simulink model "SguanFOC"  (R2025a)
settings: Solver=FixedStepAuto  StartTime=0.0  StopTime=5  FixedStep=0.00001  RelTol=1e-3
InitFcn:
  | T = 0.0001;
  | VBUS = 12;
  | 
  | Wc = 10;
  | Ws = 50;
undefined symbols (not defined in the file): Down, Up
libraries: eePwmGenerator x3, spsDCVoltageSourceLib x1, spsPermanentMagnetSynchronousMachineLib x1, spsSawtoothGeneratorLib x1, spsUniversalBridgeLib x1, spspowerguiLib x1
settings Model: Creator=星必尘Sguan  LastModifiedBy=星必尘Sguan
settings SFSimCC: SimCustomHeaderCode="#include \"SVPWM.h\""  SimUserSources=SVPWM.c

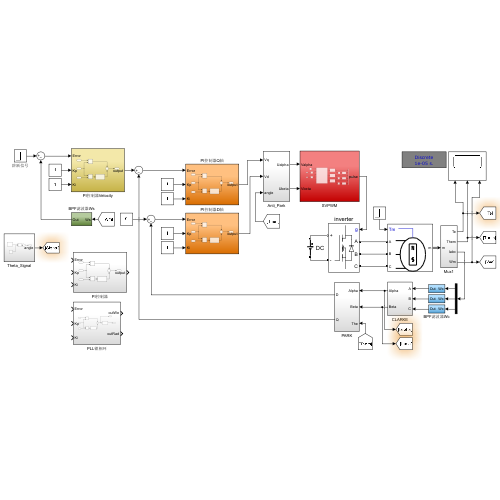
[thumbnail: Simulink's stored preview of the top-level diagram]
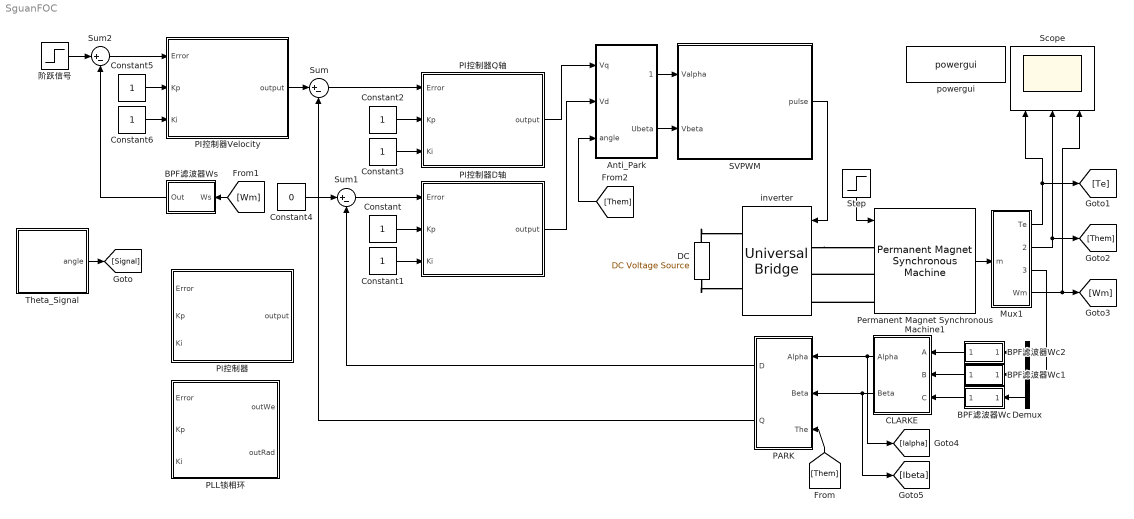
== system SguanFOC ==
  Anti_Park : Subsystem
  BPF滤波器Wc : Subsystem
  BPF滤波器Wc1 : Subsystem
  BPF滤波器Wc2 : Subsystem
  BPF滤波器Ws : Subsystem
  CLARKE : Subsystem
  Constant{,1..3,5..6} (6 alike) : Constant
  Constant4 : Constant  Value=0
  DC : spsDCVoltageSourceLib/DC Voltage Source  Amplitude=VBUS  Measurements=Voltage
  Demux : Demux  Outputs=3
  Mux1 : Subsystem
  PARK : Subsystem
  PI控制器 : Subsystem
  PI控制器D轴 : Subsystem
  PI控制器Q轴 : Subsystem
  PI控制器Velocity : Subsystem
  PLL锁相环 : Subsystem
  Permanent Magnet Synchronous Machine1 : spsPermanentMagnetSynchronousMachineLib/Permanent Magnet Synchronous Machine  NbPhases=3  FluxDistribution=Sinusoidal  RotorType=Salient-pole  MechanicalLoad=Torque Tm  PresetModel=No  ShowDetailedParameters=on  MeasurementBus=off  Resistance=0.958  Inductance=8.5e-3  dqInductances=[5.25e-3,12e-3]  La=0.000835  MachineConstant=Flux linkage established by magnets (V.s)  Flux=0.0234  VoltageCst=16.9772  TorqueCst=0.1404  Flat=120  Mechanical=[0.00025 0 4]  PolePairs=3  InitialConditions=[0,0, 0,0]  InitialConditions5ph=[0 0 0 0 0 0]  RefAngle=Aligned with phase A axis (original Park)  IterativeDiscreteModel=Trapezoidal non iterative  TsBlock=-1  TsPowergui=0
  SVPWM : Subsystem
  Scope : Scope  NumInputPorts=3
      settings: ActiveDisplayYMinimum=-17.449565790069414  ActiveDisplayYMaximum=24.577855803107717
  Step : Step  Time=0  After=0  SampleTime=0
  Sum : Sum  Inputs=|+-
  Sum1 : Sum  Inputs=|+-
  Sum2 : Sum  Inputs=|+-
  Theta_Signal : Subsystem
  inverter : spsUniversalBridgeLib/Universal Bridge  Arms=3  SnubberResistance=100  SnubberCapacitance=1e-5  Device=MOSFET / Diodes  Ron=1e-3  Lon=0  ForwardVoltages="[  0  0  ]"  ForwardVoltage=0  GTOparameters=[ 10e-6 , 20e-6 ]  IGBTparameters=[ 1e-6 , 2e-6 ]  Measurements=None  Measurements_2=None  converterType=Rectifier
  powergui : spspowerguiLib/powergui  SimulationMode=Discrete  SampleTime=1e-5  frequency=60  Iterations=50  frequencyindice=0  Pbase=100e6  ErrMax=1e-4  UnitsV=kV  UnitsW=MW  buscounter=0  FunctionMessages=off  echomessages=off  EnableUseOfTLC=off  CurrentSourceSwitches=off  DisableSnubberDevices=off  DisableRonSwitches=off  DisableVfSwitches=off  DisplayEquations=off  AutomaticDiscreteSolvers=off  SolverType=Tustin/Backward Euler (TBE)  Interpol=off  ExternalGateDelay=off  methode=off  Ts=0  x0status=blocks  SPID=off  SwTol=0  HookPort=off  NonlinearTolerance=1e-4  nMaxIteration=100  ContinueOnMaxIteration=off  RestoreLinks=warning  ResistiveCurrentMeasurement=off  Frange=[0:2:500]  Ylog=off  Xlog=on  ShowGrid=off  save=off  variable=ZData  structure=0  ZoomFFT=on  StartTime=0.0  cycles=1  DisplayStyle=1  fundamental=60  FreqAxis=off  MaxFrequency=1000  frequencyindicesteady=1  RmsSteady=1  display=off
  阶跃信号 : Step  Time=3  After=72  SampleTime=1e-5
  wires:
  Step/1 -> Permanent Magnet Synchronous Machine1/1
  Permanent Magnet Synchronous Machine1/1 -> Mux1/1(m)
  Anti_Park/1(Ualpha) -> SVPWM/1(Valpha)
  Anti_Park/2(Ubeta) -> SVPWM/2(Vbeta)
  SVPWM/1(pulse) -> inverter/1
  Mux1/3(Iabc) -> Demux/1
  Theta_Signal/1(angle) -> [Signal]
  PI控制器Q轴/1(output) -> Anti_Park/1(Vq)
  PI控制器D轴/1(output) -> Anti_Park/2(Vd)
  Constant/1 -> PI控制器D轴/2(Kp)
  Constant1/1 -> PI控制器D轴/3(Ki)
  Constant2/1 -> PI控制器Q轴/2(Kp)
  Constant3/1 -> PI控制器Q轴/3(Ki)
  Sum/1 -> PI控制器Q轴/1(Error)
  PI控制器Velocity/1(output) -> Sum/1
  Sum1/1 -> PI控制器D轴/1(Error)
  Demux/1 -> BPF滤波器Wc2/1(Wc)
  Demux/2 -> BPF滤波器Wc1/1(Wc)
  Demux/3 -> BPF滤波器Wc/1(Wc)
  CLARKE/1(Alpha) -> PARK/1(Alpha), [Ialpha]
  CLARKE/2(Beta) -> PARK/2(Beta), [Ibeta]
  Mux1/1(Te) -> [Te], Scope/1
  Mux1/2(Them) -> [Them], Scope/2
  Mux1/4(Wm) -> [Wm], Scope/3
  [Them] -> PARK/3(The)
  PARK/1(D) -> Sum1/2
  PARK/2(Q) -> Sum/2
  Constant4/1 -> Sum1/1
  阶跃信号/1 -> Sum2/1
  Sum2/1 -> PI控制器Velocity/1(Error)
  [Wm] -> BPF滤波器Ws/1(Ws)
  Constant5/1 -> PI控制器Velocity/2(Kp)
  Constant6/1 -> PI控制器Velocity/3(Ki)
  [Them] -> Anti_Park/3(angle)
  BPF滤波器Ws/1(Out) -> Sum2/2
  BPF滤波器Wc2/1(Out) -> CLARKE/1(A)
  BPF滤波器Wc1/1(Out) -> CLARKE/2(B)
  BPF滤波器Wc/1(Out) -> CLARKE/3(C)
  connections:
  DC/RConn1 -- inverter/RConn1
  DC/LConn1 -- inverter/RConn2
  inverter/LConn1 -- Permanent Magnet Synchronous Machine1/LConn1
  Permanent Magnet Synchronous Machine1/LConn2 -- inverter/LConn2
  Permanent Magnet Synchronous Machine1/LConn3 -- inverter/LConn3

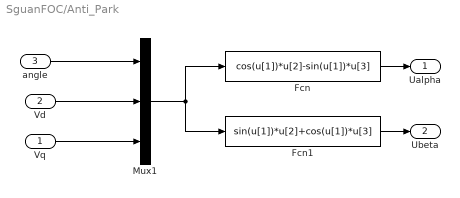
== system SguanFOC/Anti_Park ==
  Vq : Inport
  Vd : Inport  Port=2
  angle : Inport  Port=3
  Fcn : Fcn  Expr=cos(u[1])*u[2]-sin(u[1])*u[3]
  Fcn1 : Fcn  Expr=sin(u[1])*u[2]+cos(u[1])*u[3]
  Mux1 : Mux  Inputs=3
  Ualpha : Outport
  Ubeta : Outport  Port=2
  wires:
  angle/1 -> Mux1/1
  Vq/1 -> Mux1/3
  Vd/1 -> Mux1/2
  Mux1/1 -> Fcn1/1, Fcn/1
  Fcn/1 -> Ualpha/1
  Fcn1/1 -> Ubeta/1

== system SguanFOC/BPF滤波器Wc ==
  Wc : Inport
  Transfer Fcn1 : TransferFcn  Numerator=[Wc^2]  Denominator=[1 sqrt(2)*Wc Wc^2]
  Out : Outport
  wires:
  Transfer Fcn1/1 -> Out/1
  Wc/1 -> Transfer Fcn1/1

== system SguanFOC/BPF滤波器Wc1 ==
  Wc : Inport
  Transfer Fcn1 : TransferFcn  Numerator=[Wc^2]  Denominator=[1 sqrt(2)*Wc Wc^2]
  Out : Outport
  wires:
  Transfer Fcn1/1 -> Out/1
  Wc/1 -> Transfer Fcn1/1

== system SguanFOC/BPF滤波器Wc2 ==
  Wc : Inport
  Transfer Fcn1 : TransferFcn  Numerator=[Wc^2]  Denominator=[1 sqrt(2)*Wc Wc^2]
  Out : Outport
  wires:
  Transfer Fcn1/1 -> Out/1
  Wc/1 -> Transfer Fcn1/1

== system SguanFOC/BPF滤波器Ws ==
  Ws : Inport
  Transfer Fcn1 : TransferFcn  Numerator=[Ws^2]  Denominator=[1 sqrt(2)*Ws Ws^2]
  Out : Outport
  wires:
  Transfer Fcn1/1 -> Out/1
  Ws/1 -> Transfer Fcn1/1

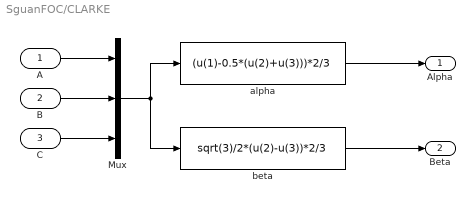
== system SguanFOC/CLARKE ==
  A : Inport
  B : Inport  Port=2
  C : Inport  Port=3
  Mux : Mux  Inputs=3
  alpha : Fcn  Expr=(u(1)-0.5*(u(2)+u(3)))*2/3
  beta : Fcn  Expr=sqrt(3)/2*(u(2)-u(3))*2/3
  Alpha : Outport
  Beta : Outport  Port=2
  wires:
  beta/1 -> Beta/1
  Mux/1 -> alpha/1, beta/1
  A/1 -> Mux/1
  C/1 -> Mux/3
  B/1 -> Mux/2
  alpha/1 -> Alpha/1

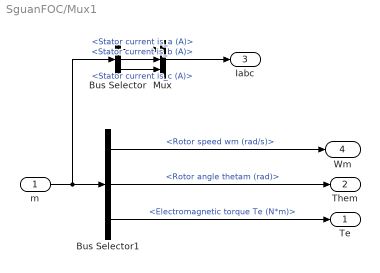
== system SguanFOC/Mux1 ==
  m : Inport
  Bus Selector : BusSelector  OutputSignals=Stator current is_a (A),Stator current is_b (A),Stator current is_c (A)
  Bus Selector1 : BusSelector  OutputSignals=Rotor speed wm (rad/s),Rotor angle thetam (rad),Electromagnetic torque Te (N*m)
  Mux : Mux  Inputs=3
  Te : Outport
  Them : Outport  Port=2
  Iabc : Outport  Port=3
  Wm : Outport  Port=4
  wires:
  Bus Selector1/2 -> Them/1  "<Rotor angle thetam (rad)>"
  Bus Selector1/3 -> Te/1  "<Electromagnetic torque Te (N*m)>"
  m/1 -> Bus Selector/1, Bus Selector1/1
  Bus Selector/2 -> Mux/2  "<Stator current is_b (A)>"
  Bus Selector/3 -> Mux/3  "<Stator current is_c (A)>"
  Bus Selector/1 -> Mux/1  "<Stator current is_a (A)>"
  Mux/1 -> Iabc/1
  Bus Selector1/1 -> Wm/1  "<Rotor speed wm (rad/s)>"

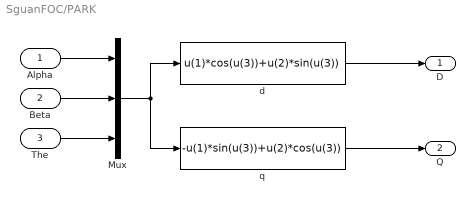
== system SguanFOC/PARK ==
  Alpha : Inport
  Beta : Inport  Port=2
  The : Inport  Port=3
  Mux : Mux  Inputs=3
  d : Fcn  Expr=u(1)*cos(u(3))+u(2)*sin(u(3))
  q : Fcn  Expr=-u(1)*sin(u(3))+u(2)*cos(u(3))
  D : Outport
  Q : Outport  Port=2
  wires:
  The/1 -> Mux/3
  q/1 -> Q/1
  Mux/1 -> d/1, q/1
  Alpha/1 -> Mux/1
  Beta/1 -> Mux/2
  d/1 -> D/1

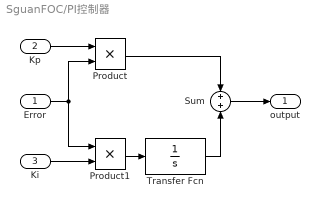
== system SguanFOC/PI控制器 ==
  Error : Inport
  Kp : Inport  Port=2
  Ki : Inport  Port=3
  Product : Product
  Product1 : Product
  Sum : Sum
  Transfer Fcn : TransferFcn  Denominator=[1 0]
  output : Outport
  wires:
  Product1/1 -> Transfer Fcn/1
  Product/1 -> Sum/1
  Ki/1 -> Product1/2
  Transfer Fcn/1 -> Sum/2
  Sum/1 -> output/1
  Error/1 -> Product1/1, Product/2
  Kp/1 -> Product/1

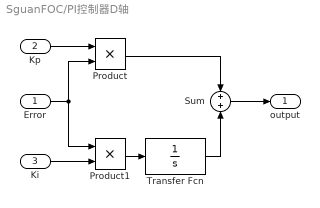
== system SguanFOC/PI控制器D轴 ==
  Error : Inport
  Kp : Inport  Port=2
  Ki : Inport  Port=3
  Product : Product
  Product1 : Product
  Sum : Sum
  Transfer Fcn : TransferFcn  Denominator=[1 0]
  output : Outport
  wires:
  Product1/1 -> Transfer Fcn/1
  Product/1 -> Sum/1
  Ki/1 -> Product1/2
  Transfer Fcn/1 -> Sum/2
  Sum/1 -> output/1
  Error/1 -> Product1/1, Product/2
  Kp/1 -> Product/1

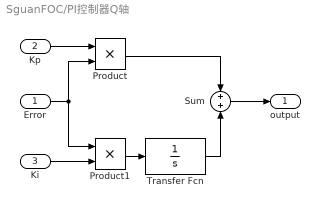
== system SguanFOC/PI控制器Q轴 ==
  Error : Inport
  Kp : Inport  Port=2
  Ki : Inport  Port=3
  Product : Product
  Product1 : Product
  Sum : Sum
  Transfer Fcn : TransferFcn  Denominator=[1 0]
  output : Outport
  wires:
  Product1/1 -> Transfer Fcn/1
  Product/1 -> Sum/1
  Ki/1 -> Product1/2
  Transfer Fcn/1 -> Sum/2
  Sum/1 -> output/1
  Error/1 -> Product1/1, Product/2
  Kp/1 -> Product/1

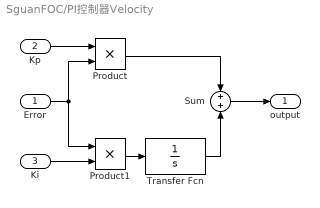
== system SguanFOC/PI控制器Velocity ==
  Error : Inport
  Kp : Inport  Port=2
  Ki : Inport  Port=3
  Product : Product
  Product1 : Product
  Sum : Sum
  Transfer Fcn : TransferFcn  Denominator=[1 0]
  output : Outport
  wires:
  Product1/1 -> Transfer Fcn/1
  Product/1 -> Sum/1
  Ki/1 -> Product1/2
  Transfer Fcn/1 -> Sum/2
  Sum/1 -> output/1
  Error/1 -> Product1/1, Product/2
  Kp/1 -> Product/1

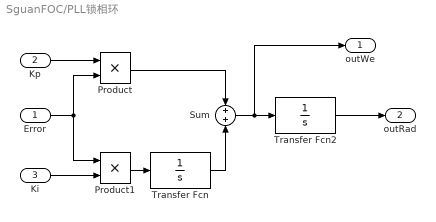
== system SguanFOC/PLL锁相环 ==
  Error : Inport
  Kp : Inport  Port=2
  Ki : Inport  Port=3
  Product : Product
  Product1 : Product
  Sum : Sum
  Transfer Fcn : TransferFcn  Denominator=[1 0]
  Transfer Fcn2 : TransferFcn  Denominator=[1 0]
  outWe : Outport
  outRad : Outport  Port=2
  wires:
  Product/1 -> Sum/1
  Sum/1 -> outWe/1, Transfer Fcn2/1
  Error/1 -> Product1/1, Product/2
  Transfer Fcn2/1 -> outRad/1
  Transfer Fcn/1 -> Sum/2
  Ki/1 -> Product1/2
  Product1/1 -> Transfer Fcn/1
  Kp/1 -> Product/1

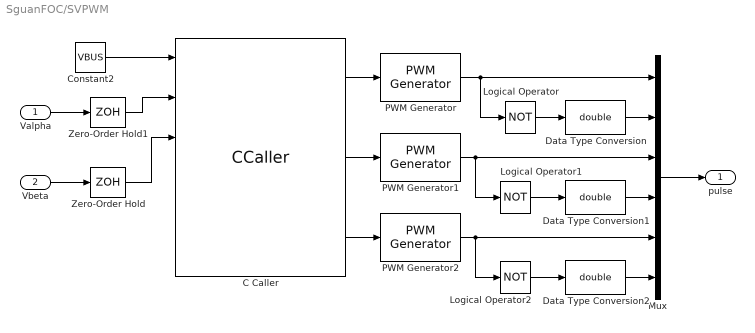
== system SguanFOC/SVPWM ==
  Valpha : Inport
  Vbeta : Inport  Port=2
  C Caller : CCaller  FunctionName=SVPWM  PortSpecificationStruct="%)30     .    8 H   8    (     @         %    \"     8    !     0         %  0 \"0    $    _    07)G3F%M90  4&]R=$YA;64 4V-O<&4     26YD97@     5'EP90      4VEZ90      27-';&]B86P   X    P    !@    @    $          4    (     0    0    !         !  ! !60E53#@   #     &    \"     0         !0    @    !    !     $         $  $ %9\"55,.    .     8    (    !          %    \"     $    %     0         0  ...(+3198 chars)"
  Constant2 : Constant  Value=VBUS
  Data Type Conversion : DataTypeConversion  OutDataTypeStr=double  SaturateOnIntegerOverflow=off  RndMeth=Floor
  Data Type Conversion1 : DataTypeConversion  OutDataTypeStr=double  SaturateOnIntegerOverflow=off  RndMeth=Floor
  Data Type Conversion2 : DataTypeConversion  OutDataTypeStr=double  SaturateOnIntegerOverflow=off  RndMeth=Floor
  Logical Operator : Logic  Operator=NOT  AllPortsSameDT=off  OutDataTypeStr=boolean
  Logical Operator1 : Logic  Operator=NOT  AllPortsSameDT=off  OutDataTypeStr=boolean
  Logical Operator2 : Logic  Operator=NOT  AllPortsSameDT=off  OutDataTypeStr=boolean
  Mux : Mux  Inputs=6
  PWM Generator : eePwmGenerator/PWM Generator  CarrCount=Up-Down  Tper=0.0001  Tdelay=0  Ts=1e-5
  PWM Generator1 : eePwmGenerator/PWM Generator  CarrCount=Up-Down  Tper=0.0001  Tdelay=0  Ts=1e-5
  PWM Generator2 : eePwmGenerator/PWM Generator  CarrCount=Up-Down  Tper=0.0001  Tdelay=0  Ts=1e-5
  Zero-Order Hold : ZeroOrderHold  SampleTime=T
  Zero-Order Hold1 : ZeroOrderHold  SampleTime=T
  pulse : Outport
  wires:
  Data Type Conversion2/1 -> Mux/6
  Logical Operator2/1 -> Data Type Conversion2/1
  PWM Generator/1 -> Mux/1, Logical Operator/1
  C Caller/1 -> PWM Generator/1
  Logical Operator1/1 -> Data Type Conversion1/1
  Constant2/1 -> C Caller/1
  Zero-Order Hold1/1 -> C Caller/2
  Data Type Conversion/1 -> Mux/2
  Data Type Conversion1/1 -> Mux/4
  Mux/1 -> pulse/1
  Zero-Order Hold/1 -> C Caller/3
  PWM Generator2/1 -> Logical Operator2/1, Mux/5
  PWM Generator1/1 -> Logical Operator1/1, Mux/3
  Logical Operator/1 -> Data Type Conversion/1
  Vbeta/1 -> Zero-Order Hold/1
  C Caller/2 -> PWM Generator1/1
  C Caller/3 -> PWM Generator2/1
  Valpha/1 -> Zero-Order Hold1/1

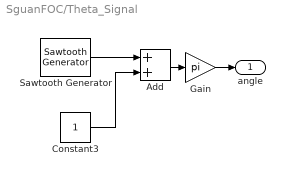
== system SguanFOC/Theta_Signal ==
  Add : Sum
  Constant3 : Constant
  Gain : Gain  Gain=pi
  Sawtooth Generator : spsSawtoothGeneratorLib/Sawtooth Generator  Freq=1  Phase=180  Ts=0
  angle : Outport
  wires:
  Add/1 -> Gain/1
  Constant3/1 -> Add/2
  Gain/1 -> angle/1
  Sawtooth Generator/1 -> Add/1
